simulink model "Third3"  (R2017b)
settings: Solver=VariableStepAuto  StartTime=0.0  StopTime=10.0  RelTol=1e-3
settings Model: Creator=17863  LastModifiedBy=17863

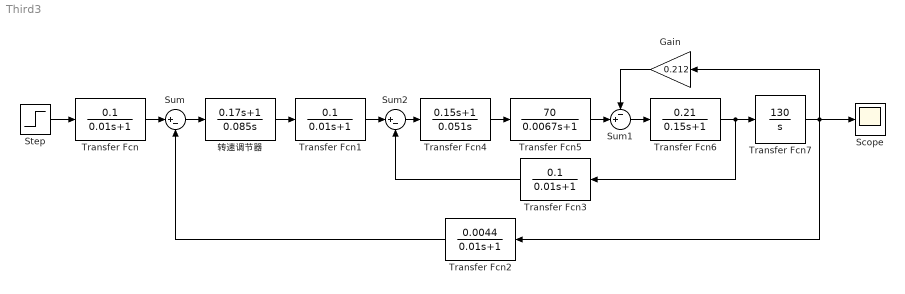
== system Third3 ==
  Gain : Gain  Gain=0.212
  Scope : Scope
  Step : Step  SampleTime=0
  Sum : Sum  Inputs=|+-
  Sum1 : Sum  Inputs=-+|
  Sum2 : Sum  Inputs=|+-
  Transfer Fcn : TransferFcn  Numerator=[0.1]  Denominator=[0.01 1]
  Transfer Fcn1 : TransferFcn  Numerator=[0.1]  Denominator=[0.01 1]
  Transfer Fcn2 : TransferFcn  Numerator=[0.0044]  Denominator=[0.01 1]
  Transfer Fcn3 : TransferFcn  Numerator=[0.1]  Denominator=[0.01 1]
  Transfer Fcn4 : TransferFcn  Numerator=[0.15 1]  Denominator=[0.051 0]
  Transfer Fcn5 : TransferFcn  Numerator=[70]  Denominator=[0.0067 1]
  Transfer Fcn6 : TransferFcn  Numerator=[0.21]  Denominator=[0.15 1]
  Transfer Fcn7 : TransferFcn  Numerator=[130]  Denominator=[1 0]
  "转速调节器 " : TransferFcn  Numerator=[0.17 1]  Denominator=[0.085 0]
  wires:
  Step/1 -> Transfer Fcn/1
  Transfer Fcn/1 -> Sum/1
  Sum/1 -> "转速调节器 "/1
  "转速调节器 "/1 -> Transfer Fcn1/1
  Transfer Fcn1/1 -> Sum2/1
  Sum2/1 -> Transfer Fcn4/1
  Transfer Fcn4/1 -> Transfer Fcn5/1
  Transfer Fcn5/1 -> Sum1/2
  Gain/1 -> Sum1/1
  Sum1/1 -> Transfer Fcn6/1
  Transfer Fcn6/1 -> Transfer Fcn3/1, Transfer Fcn7/1
  Transfer Fcn7/1 -> Transfer Fcn2/1, Gain/1, Scope/1
  Transfer Fcn3/1 -> Sum2/2
  Transfer Fcn2/1 -> Sum/2
